simulink model "System_Identification"  (R2019a)
settings: Solver=FixedStepAuto  StartTime=0.0  StopTime=10.0  FixedStep=1e-3  RelTol=1e-3
libraries: simulink x1, cstblocks x1
settings Model: Creator=capn  LastModifiedBy=emma
settings DataIOCC: ReturnWorkspaceOutputs=off
settings DebuggingCC: ArithmeticOperatorsInVariantConditions=warning
settings SFSimCC: SimUseLocalCustomCode=off
settings RTWCC: RTWUseLocalCustomCode=off
settings CodeAppCC: StateflowObjectComments=on

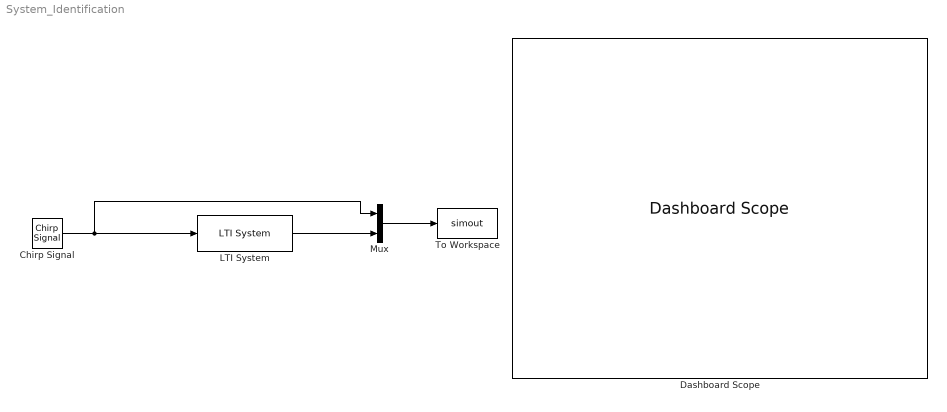
== system System_Identification ==
  Chirp Signal : simulink/Sources/Chirp Signal  f1=0.1  T=10  f2=100
  Dashboard Scope : DashboardScope
  LTI System : cstblocks/LTI System  sys=tf(1,[1 1 5])  IC=[]
  Mux : Mux  Inputs=2
  To Workspace : ToWorkspace  VariableName=simout  SampleTime=-1
  wires:
  Chirp Signal/1 -> LTI System/1, Mux/1
  LTI System/1 -> Mux/2
  Mux/1 -> To Workspace/1
